simulink model "DiscreteControllerR2024"  (R2025a)
settings: Solver=ode1  StartTime=0.0  StopTime=30  FixedStep=0.002  RelTol=1e-3
values from neighbouring files (symbols this model uses):
  A = [ -0.6 -0.76 0    0 ... (first row only)    [aircraft_flare_lqr_observer.m]
  A12 = ss_new.A(1:p,p+1:n)    [aircraft_flare_lqr_observer.m]
  A21 = ss_new.A(p+1:n,1:p)    [aircraft_flare_lqr_observer.m]
  Ad = ss_new.A(p+1:n,p+1:n)    [aircraft_flare_lqr_observer.m]
  B = [ -2.375; 0; 0; 0 ]    [aircraft_flare_lqr_observer.m]
  Bd = ss_new.B(p+1:n,1:m)    [aircraft_flare_lqr_observer.m]
  C = [ 1 0 0 0 ... (first row only)    [aircraft_flare_lqr_observer.m]
  D = 0    [aircraft_flare_lqr_observer.m]
  IC_PLANT = X0(i,:)    [aircraft_flare_lqr_observer.m]
  IC_X_HAT = 256*X0(i,2)    [aircraft_flare_lqr_observer.m]
  K = lqr(A,B,Q,R)    [aircraft_flare_lqr_observer.m]
  Kr = [K(3) K(4)]    [aircraft_flare_lqr_observer.m]
  L = L'    [aircraft_flare_lqr_observer.m]
  T = [C;[0 0 1 0]]    [aircraft_flare_lqr_observer.m]
settings Model: Creator=gui  LastModifiedBy=gui
settings DebuggingCC: AlgebraicLoopMsg=none

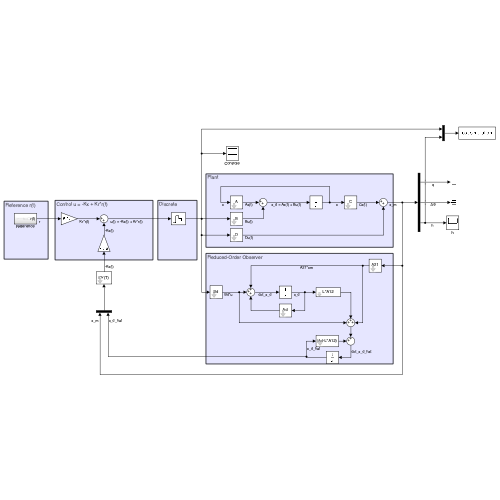
[thumbnail: Simulink's stored preview of the top-level diagram]
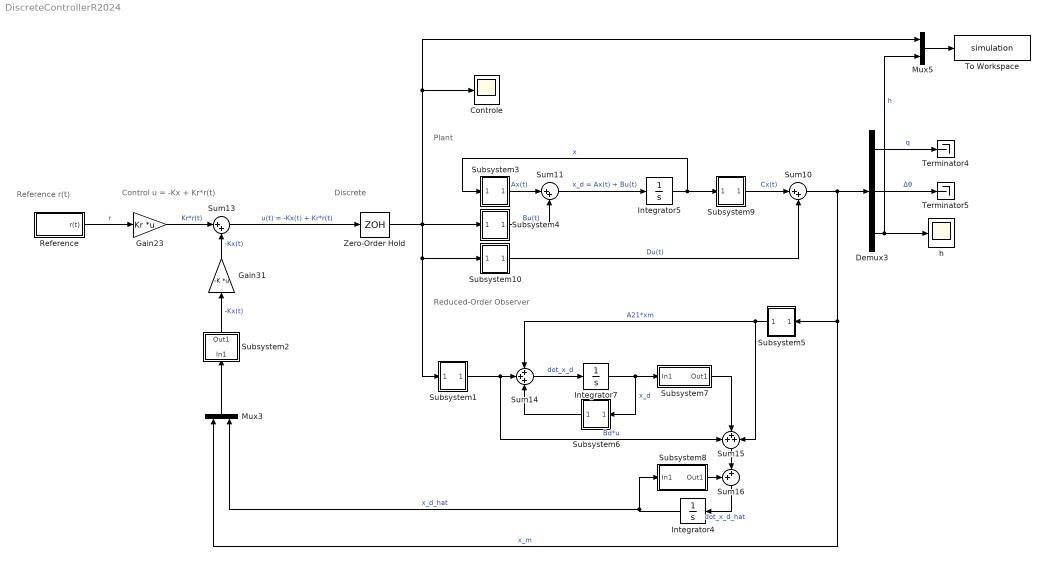
== system DiscreteControllerR2024 ==
  note: Reduced-Order Observer
  note: Control u = -Kx + Kr*r(t)
  note: Plant
  note: Reference r(t)
  note: Discrete
  Controle : Scope
      settings: ActiveDisplayYMinimum=-21.1446  ActiveDisplayYMaximum=113.4605  DataLoggingVariableName=ScopeData3
  Demux3 : Demux  Outputs=3
  Gain23 : Gain  Gain=Kr  Multiplication=Matrix(K*u)
  Gain31 : Gain  Gain=-K  Multiplication=Matrix(K*u)
  Integrator4 : Integrator  InitialCondition=IC_X_HAT
  Integrator5 : Integrator  InitialCondition=IC_PLANT
  Integrator7 : Integrator  InitialCondition=IC_X_HAT
  Mux3 : Mux  Inputs=2
  Mux5 : Mux  Inputs=2
  Reference : Subsystem
  Subsystem1 : Subsystem  mask{K=Bd}
      mask prompts: K "Gain"
      mask Display:
      | gainStr = get_param(gcb, 'K');
      | disp(gainStr);
  Subsystem10 : Subsystem  mask{K=D}
      mask prompts: K "Gain"
      mask Display:
      | gainStr = get_param(gcb, 'K');
      | disp(gainStr);
  Subsystem2 : Subsystem  mask{K=inv(T)}
      mask prompts: K "Gain"
      mask Display:
      | gainStr = get_param(gcb, 'K');
      | disp(gainStr);
  Subsystem3 : Subsystem  mask{K=A}
      mask prompts: K "Gain"
      mask Display:
      | gainStr = get_param(gcb, 'K');
      | disp(gainStr);
  Subsystem4 : Subsystem  mask{K=B}
      mask prompts: K "Gain"
      mask Display:
      | gainStr = get_param(gcb, 'K');
      | disp(gainStr);
  Subsystem5 : Subsystem  mask{K=A21}
      mask prompts: K "Gain"
      mask Display:
      | gainStr = get_param(gcb, 'K');
      | disp(gainStr);
  Subsystem6 : Subsystem  mask{K=Ad}
      mask prompts: K "Gain"
      mask Display:
      | gainStr = get_param(gcb, 'K');
      | disp(gainStr);
  Subsystem7 : Subsystem  mask{K=L*A12}
      mask prompts: K "Gain"
      mask Display:
      | gainStr = get_param(gcb, 'K');
      | disp(gainStr);
  Subsystem8 : Subsystem  mask{K=(Ad-L*A12)}
      mask prompts: K "Gain"
      mask Display:
      | gainStr = get_param(gcb, 'K');
      | disp(gainStr);
  Subsystem9 : Subsystem  mask{K=C}
      mask prompts: K "Gain"
      mask Display:
      | gainStr = get_param(gcb, 'K');
      | disp(gainStr);
  Sum10 : Sum  Inputs=|++
  Sum11 : Sum  Inputs=|++
  Sum13 : Sum  Inputs=|++
  Sum14 : Sum  Inputs=+++
  Sum15 : Sum  Inputs=+++
  Sum16 : Sum  Inputs=++|
  Terminator4 : Terminator
  Terminator5 : Terminator
  To Workspace : ToWorkspace  VariableName=simulation  SaveFormat=Structure With Time  SampleTime=-1
  Zero-Order Hold : ZeroOrderHold  SampleTime=0.2
  h : Scope
      settings: ActiveDisplayYMinimum=-17.7112  ActiveDisplayYMaximum=90.8568  DataLoggingVariableName=ScopeData4
  wires:
  Subsystem2/1(Out1) -> Gain31/1  "-Kx(t)"
  Gain31/1 -> Sum13/2  "-Kx(t)"
  Sum11/1 -> Integrator5/1  "x_d = Ax(t) + Bu(t)"
  Subsystem4/1(Out1) -> Sum11/2  "Bu(t)"
  Subsystem3/1(Out1) -> Sum11/1  "Ax(t)"
  Demux3/1 -> Terminator4/1  "q"
  Sum10/1 -> Subsystem5/1(In1), Mux3/1, Demux3/1  "x_m"
  Mux5/1 -> To Workspace/1
  Subsystem10/1(Out1) -> Sum10/2  "Du(t)"
  Sum13/1 -> Zero-Order Hold/1  "u(t) = -Kx(t) + Kr*r(t)"
  Reference/1(r(t)) -> Gain23/1  "r"
  Demux3/2 -> Terminator5/1  "Δθ"
  Gain23/1 -> Sum13/1  "Kr*r(t)"
  Integrator5/1 -> Subsystem9/1(In1), Subsystem3/1(In1)  "x"
  Subsystem9/1(Out1) -> Sum10/1  "Cx(t)"
  Demux3/3 -> Mux5/2, h/1  "h"
  Mux3/1 -> Subsystem2/1(In1)
  Zero-Order Hold/1 -> Subsystem4/1(In1), Subsystem10/1(In1), Subsystem1/1(In1), Controle/1, Mux5/1
  Subsystem1/1(Out1) -> Sum15/1, Sum14/2  "Bd*u"
  Subsystem5/1(Out1) -> Sum15/3, Sum14/1  "A21*xm"
  Sum14/1 -> Integrator7/1  "dot_x_d"
  Integrator7/1 -> Subsystem7/1(In1), Subsystem6/1(In1)  "x_d"
  Subsystem6/1(Out1) -> Sum14/3
  Subsystem7/1(Out1) -> Sum15/2
  Sum16/1 -> Integrator4/1  "dot_x_d_hat"
  Sum15/1 -> Sum16/2
  Subsystem8/1(Out1) -> Sum16/1
  Integrator4/1 -> Mux3/2, Subsystem8/1(In1)  "x_d_hat"

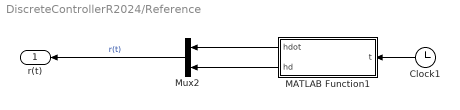
== system DiscreteControllerR2024/Reference ==
  Clock1 : Clock
  MATLAB Function1 : MATLAB Function  TreatAsAtomicUnit=on
  Mux2 : Mux  Inputs=2
  r(t) : Outport
  wires:
  MATLAB Function1/2(hd) -> Mux2/2
  Mux2/1 -> r(t)/1  "r(t)"
  Clock1/1 -> MATLAB Function1/1(t)
  MATLAB Function1/1(hdot) -> Mux2/1

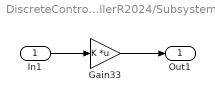
== system DiscreteControllerR2024/Subsystem1 ==
  In1 : Inport
  Gain33 : Gain  Gain=K  Multiplication=Matrix(K*u)
  Out1 : Outport
  wires:
  In1/1 -> Gain33/1
  Gain33/1 -> Out1/1

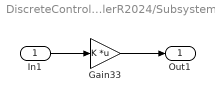
== system DiscreteControllerR2024/Subsystem10 ==
  In1 : Inport
  Gain33 : Gain  Gain=K  Multiplication=Matrix(K*u)
  Out1 : Outport
  wires:
  In1/1 -> Gain33/1
  Gain33/1 -> Out1/1

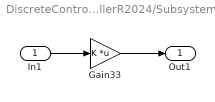
== system DiscreteControllerR2024/Subsystem2 ==
  In1 : Inport
  Gain33 : Gain  Gain=K  Multiplication=Matrix(K*u)
  Out1 : Outport
  wires:
  In1/1 -> Gain33/1
  Gain33/1 -> Out1/1

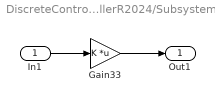
== system DiscreteControllerR2024/Subsystem3 ==
  In1 : Inport
  Gain33 : Gain  Gain=K  Multiplication=Matrix(K*u)
  Out1 : Outport
  wires:
  In1/1 -> Gain33/1
  Gain33/1 -> Out1/1

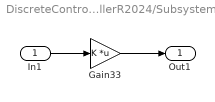
== system DiscreteControllerR2024/Subsystem4 ==
  In1 : Inport
  Gain33 : Gain  Gain=K  Multiplication=Matrix(K*u)
  Out1 : Outport
  wires:
  In1/1 -> Gain33/1
  Gain33/1 -> Out1/1

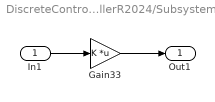
== system DiscreteControllerR2024/Subsystem5 ==
  In1 : Inport
  Gain33 : Gain  Gain=K  Multiplication=Matrix(K*u)
  Out1 : Outport
  wires:
  In1/1 -> Gain33/1
  Gain33/1 -> Out1/1

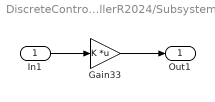
== system DiscreteControllerR2024/Subsystem6 ==
  In1 : Inport
  Gain33 : Gain  Gain=K  Multiplication=Matrix(K*u)
  Out1 : Outport
  wires:
  In1/1 -> Gain33/1
  Gain33/1 -> Out1/1

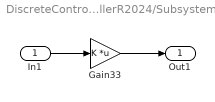
== system DiscreteControllerR2024/Subsystem7 ==
  In1 : Inport
  Gain33 : Gain  Gain=K  Multiplication=Matrix(K*u)
  Out1 : Outport
  wires:
  In1/1 -> Gain33/1
  Gain33/1 -> Out1/1

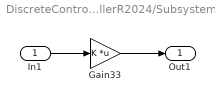
== system DiscreteControllerR2024/Subsystem8 ==
  In1 : Inport
  Gain33 : Gain  Gain=K  Multiplication=Matrix(K*u)
  Out1 : Outport
  wires:
  In1/1 -> Gain33/1
  Gain33/1 -> Out1/1

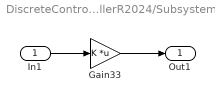
== system DiscreteControllerR2024/Subsystem9 ==
  In1 : Inport
  Gain33 : Gain  Gain=K  Multiplication=Matrix(K*u)
  Out1 : Outport
  wires:
  In1/1 -> Gain33/1
  Gain33/1 -> Out1/1

== matlab function DiscreteControllerR2024/Reference/MATLAB Function1 ==
  data: t input; hdot output; hd output
function [hdot, hd] = r(t)
%#codegen
% Gera h_d(t) e hdot_d(t)

if t <= 15
    hd   = 100*exp(-t/5);
    hdot = -20*exp(-t/5);   % derivada de 100*exp(-t/5)
else
    hd   = 20 - t;
    hdot = -1;              % derivada de (20 - t)
end
